simulink model "neural_hopper_wetrace_TD"  (R2018a)
settings: Solver=ode45  StartTime=0.0  StopTime=20  RelTol=1e-4  AbsTol=1e-6  EnableMultiTasking=on
values from neighbouring files (symbols this model uses):
  a = 10    [neural_hopper_wetrace_ISO_params.m]    (also in neural_hopper_wetrace_TD_params.m; neural_hopper_wetrace_params.m)
  b = 10    [neural_hopper_wetrace_ISO_params.m]    (also in neural_hopper_wetrace_TD_params.m; neural_hopper_wetrace_params.m)
  bE = 2.5    [neural_hopper_diff_hebb_params.m]    (also in neural_hopper_params.m = 0.1; neural_hopper_wetrace_ISO_params.m = 0.1; neural_hopper_wetrace_TD_params.m = 0.1; neural_hopper_wetrace_params.m = 0.1)
  c = 0.05    [neural_hopper_diff_hebb_params.m]    (also in neural_hopper_params.m; neural_hopper_wetrace_ISO_params.m; neural_hopper_wetrace_TD_params.m; neural_hopper_wetrace_params.m)
  c_w_F = 0.15    [neural_hopper_wetrace_ISO_params.m]    (also in neural_hopper_wetrace_TD_params.m)
  c_w_l = 0.15    [neural_hopper_wetrace_ISO_params.m]    (also in neural_hopper_wetrace_TD_params.m)
  c_w_v = 0.15    [neural_hopper_wetrace_ISO_params.m]    (also in neural_hopper_wetrace_TD_params.m)
  dy0 = 0    [neural_hopper_diff_hebb_params.m]    (also in neural_hopper_params.m; neural_hopper_wetrace_ISO_params.m; neural_hopper_wetrace_TD_params.m; neural_hopper_wetrace_params.m)
  eref = 0.04    [neural_hopper_diff_hebb_params.m]    (also in neural_hopper_params.m; neural_hopper_wetrace_ISO_params.m; neural_hopper_wetrace_TD_params.m; neural_hopper_wetrace_params.m)
  FmaxVAS = 22000    [neural_hopper_diff_hebb_params.m]    (also in neural_hopper_params.m; neural_hopper_wetrace_ISO_params.m; neural_hopper_wetrace_TD_params.m; neural_hopper_wetrace_params.m)
  g = 9.81    [neural_hopper_diff_hebb_params.m]    (also in neural_hopper_params.m; neural_hopper_wetrace_ISO_params.m; neural_hopper_wetrace_TD_params.m; neural_hopper_wetrace_params.m)
  G_F = 1/(N*FmaxVAS)    (= 3.0303030303e-05)    [neural_hopper_diff_hebb_params.m]    (also in neural_hopper_params.m; neural_hopper_wetrace_ISO_params.m; neural_hopper_wetrace_TD_params.m; neural_hopper_wetrace_params.m)
  G_l = 1/loptVAS    (= 10)    [neural_hopper_diff_hebb_params.m]    (also in neural_hopper_params.m; neural_hopper_wetrace_ISO_params.m = 5; neural_hopper_wetrace_TD_params.m = 5; neural_hopper_wetrace_params.m)
  G_v = -1/(vmaxVAS*loptVAS)    (= -0.833333333333)    [neural_hopper_diff_hebb_params.m]    (also in neural_hopper_params.m; neural_hopper_wetrace_ISO_params.m = -0.416666666667; neural_hopper_wetrace_TD_params.m = -0.416666666667; neural_hopper_wetrace_params.m)
  K = 5    [neural_hopper_diff_hebb_params.m]    (also in neural_hopper_params.m; neural_hopper_wetrace_ISO_params.m; neural_hopper_wetrace_TD_params.m; neural_hopper_wetrace_params.m)
  K_F_et = 200    [neural_hopper_wetrace_ISO_params.m]    (also in neural_hopper_wetrace_TD_params.m; neural_hopper_wetrace_params.m)
  K_l_et = 200    [neural_hopper_wetrace_ISO_params.m]    (also in neural_hopper_wetrace_TD_params.m; neural_hopper_wetrace_params.m)
  K_v_et = 200    [neural_hopper_wetrace_ISO_params.m]    (also in neural_hopper_wetrace_TD_params.m; neural_hopper_wetrace_params.m)
  l0 = 0.99    [neural_hopper_diff_hebb_params.m]    (also in neural_hopper_params.m = 0.9; neural_hopper_wetrace_ISO_params.m; neural_hopper_wetrace_TD_params.m; neural_hopper_wetrace_params.m = 0.9)
  loptVAS = 0.1    [neural_hopper_diff_hebb_params.m]    (also in neural_hopper_params.m; neural_hopper_wetrace_ISO_params.m; neural_hopper_wetrace_TD_params.m; neural_hopper_wetrace_params.m)
  ls = 0.5    [neural_hopper_diff_hebb_params.m]    (also in neural_hopper_params.m; neural_hopper_wetrace_ISO_params.m; neural_hopper_wetrace_TD_params.m; neural_hopper_wetrace_params.m)
  lslackVAS = 0.4    [neural_hopper_diff_hebb_params.m]    (also in neural_hopper_params.m; neural_hopper_wetrace_ISO_params.m; neural_hopper_wetrace_TD_params.m; neural_hopper_wetrace_params.m)
  lVAS0 = loptVAS+lslackVAS    (= 0.5)    [neural_hopper_diff_hebb_params.m]    (also in neural_hopper_params.m; neural_hopper_wetrace_ISO_params.m; neural_hopper_wetrace_TD_params.m; neural_hopper_wetrace_params.m)
  m = 80    [neural_hopper_diff_hebb_params.m]    (also in neural_hopper_params.m; neural_hopper_wetrace_ISO_params.m; neural_hopper_wetrace_TD_params.m; neural_hopper_wetrace_params.m)
  N = 1.5    [neural_hopper_diff_hebb_params.m]    (also in neural_hopper_params.m; neural_hopper_wetrace_ISO_params.m; neural_hopper_wetrace_TD_params.m; neural_hopper_wetrace_params.m)
  r0 = 0.05    [neural_hopper_diff_hebb_params.m]    (also in neural_hopper_params.m; neural_hopper_wetrace_ISO_params.m; neural_hopper_wetrace_TD_params.m; neural_hopper_wetrace_params.m)
  tau = 0.01    [neural_hopper_diff_hebb_params.m]    (also in neural_hopper_params.m; neural_hopper_wetrace_ISO_params.m; neural_hopper_wetrace_TD_params.m; neural_hopper_wetrace_params.m)
  tau_E = 12    [neural_hopper_diff_hebb_params.m]    (also in neural_hopper_params.m; neural_hopper_wetrace_ISO_params.m; neural_hopper_wetrace_TD_params.m; neural_hopper_wetrace_params.m)
  tauE = 0.01    [neural_hopper_diff_hebb_params.m]    (also in neural_hopper_params.m; neural_hopper_wetrace_ISO_params.m; neural_hopper_wetrace_TD_params.m; neural_hopper_wetrace_params.m)
  tauW = 50    [neural_hopper_diff_hebb_params.m]    (also in neural_hopper_params.m = 0.1; neural_hopper_wetrace_ISO_params.m = 0.01; neural_hopper_wetrace_TD_params.m = 0.035; neural_hopper_wetrace_params.m = 0.1)
  theta_u = zeros(3,1)    [neural_hopper_diff_hebb_params.m]    (also in neural_hopper_params.m; neural_hopper_wetrace_ISO_params.m = [0;0;0;0]; neural_hopper_wetrace_TD_params.m = [0;0;0]; neural_hopper_wetrace_params.m)
  thetak0 = 110*pi/180    (= 1.91986217719)    [neural_hopper_diff_hebb_params.m]    (also in neural_hopper_params.m; neural_hopper_wetrace_ISO_params.m; neural_hopper_wetrace_TD_params.m; neural_hopper_wetrace_params.m)
  v_offset = 0    [neural_hopper_wetrace_ISO_params.m]    (also in neural_hopper_wetrace_TD_params.m)
  vmaxVAS = 12    [neural_hopper_diff_hebb_params.m]    (also in neural_hopper_params.m; neural_hopper_wetrace_ISO_params.m; neural_hopper_wetrace_TD_params.m; neural_hopper_wetrace_params.m)
  w = 0.4    [neural_hopper_diff_hebb_params.m]    (also in neural_hopper_params.m; neural_hopper_wetrace_ISO_params.m; neural_hopper_wetrace_TD_params.m; neural_hopper_wetrace_params.m)
  w_F_0 = w_f(3)    [neural_hopper_diff_hebb_params.m]    (also in neural_hopper_params.m = 1; neural_hopper_wetrace_ISO_params.m = 1; neural_hopper_wetrace_TD_params.m = 1; neural_hopper_wetrace_params.m)
  w_F_upper = 4    [neural_hopper_wetrace_ISO_params.m]    (also in neural_hopper_wetrace_TD_params.m)
  w_l_0 = w_f(1)    [neural_hopper_diff_hebb_params.m]    (also in neural_hopper_params.m = 1; neural_hopper_wetrace_ISO_params.m = 1; neural_hopper_wetrace_TD_params.m = 1; neural_hopper_wetrace_params.m)
  w_l_upper = 4    [neural_hopper_wetrace_ISO_params.m]    (also in neural_hopper_wetrace_TD_params.m)
  w_v_0 = w_f(2)    [neural_hopper_diff_hebb_params.m]    (also in neural_hopper_params.m = 1; neural_hopper_wetrace_ISO_params.m = 1; neural_hopper_wetrace_TD_params.m = 1; neural_hopper_wetrace_params.m)
  w_v_upper = 4    [neural_hopper_wetrace_ISO_params.m]    (also in neural_hopper_wetrace_TD_params.m)
  y0 = l0+0.2    (= 1.19)    [neural_hopper_diff_hebb_params.m]    (also in neural_hopper_params.m = 1.1; neural_hopper_wetrace_ISO_params.m; neural_hopper_wetrace_TD_params.m; neural_hopper_wetrace_params.m = 1.1)
libraries: simulink_extras x2, simulink x1
settings Model: Creator=hgeyer  LastModifiedBy=ashwin
settings SolverCC: AutoScaleAbsTol=off
settings DataIOCC: LimitDataPoints=on  SaveFormat=Array  SignalLoggingSaveFormat=ModelDataLogs
settings OptimizationCC: ExpressionDepthLimit=2147483647  LifeSpan=inf
settings DebuggingCC: UnderspecifiedInitializationDetection=Classic  MergeDetectMultiDrivingBlocksExec=none  SolverPrmCheckMsg=warning  FcnCallInpInsideContextMsg=warning  StateNameClashWarn=warning  SFUnexpectedBacktrackingDiag=warning  SFNoUnconditionalDefaultTransitionDiag=warning  SFExecutionAtInitializationDiag=none
settings HardwareCC: ProdBitPerPointer=32  ProdBitPerSizeT=32  ProdBitPerPtrDiffT=32  ProdLargestAtomicFloat=None  ProdIntDivRoundTo=Undefined  ProdEndianess=Unspecified  ProdWordSize=32  ProdHWDeviceType=32-bit Generic
settings ModelReferenceCC: PropagateSignalLabelsOutOfModel=off
settings CodeAppCC: StateflowObjectComments=on
settings GRTTargetCC: TargetLangStandard=C89/C90 (ANSI)  GeneratePreprocessorConditionals=Disable all
settings ConfigComp: CovMetricSettings=dw  CovHtmlReporting=on  CovSaveCumulativeToWorkspaceVar=on  CovSaveSingleToWorkspaceVar=on  CovExternalEMLEnable=off

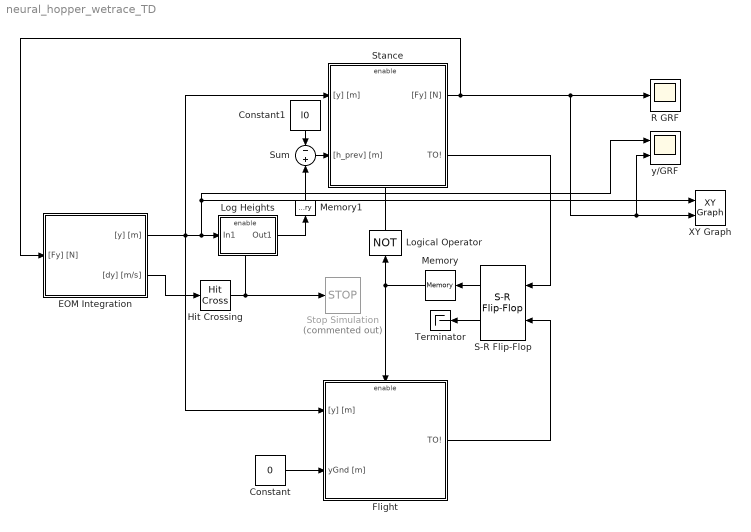
== system neural_hopper_wetrace_TD ==
  Constant : Constant  Value=0
  Constant1 : Constant  Value=l0
  EOM Integration : Subsystem
  Flight : Subsystem
  Hit Crossing : HitCross  HitCrossingDirection=falling
  Log Heights : Subsystem
  Logical Operator : Logic  Operator=NOT  AllPortsSameDT=off  OutDataTypeStr=boolean
  Memory : Memory  InitialCondition=1
  Memory1 : Memory  InitialCondition=y0
  R GRF : Scope
  S-R Flip-Flop : simulink_extras/Flip Flops/S-R Flip-Flop  initial_condition=1
  Stance : Subsystem
  Stop Simulation : Stop  Commented=on
  Sum : Sum  Inputs=-+
  Terminator : Terminator
  XY Graph : simulink/Sinks/XY Graph  xmin=0.6  xmax=1  ymin=0  ymax=5000  st=-1
  "y/GRF " : Scope  NumInputPorts=2
  wires:
  EOM Integration/1("[y] [m]") -> Log Heights/1(In1), "y/GRF "/1, XY Graph/1, Flight/1("[y] [m]"), Stance/1("[y] [m]")
  Stance/2(TO!) -> S-R Flip-Flop/1
  S-R Flip-Flop/1 -> Memory/1
  Logical Operator/1 -> Stance/Enable
  Memory/1 -> Logical Operator/1, Flight/Enable
  Flight/1(TO!) -> S-R Flip-Flop/2
  S-R Flip-Flop/2 -> Terminator/1
  Stance/1("[Fy] [N]") -> "y/GRF "/2, XY Graph/2, R GRF/1, EOM Integration/1("[Fy] [N]")
  Constant/1 -> Flight/2(yGnd [m])
  EOM Integration/2("[dy] [m/s]") -> Hit Crossing/1
  Hit Crossing/1 -> Stop Simulation/1, Log Heights/Enable
  Sum/1 -> Stance/2("[h_prev] [m]")
  Log Heights/1(Out1) -> Memory1/1
  Constant1/1 -> Sum/1
  Memory1/1 -> Sum/2

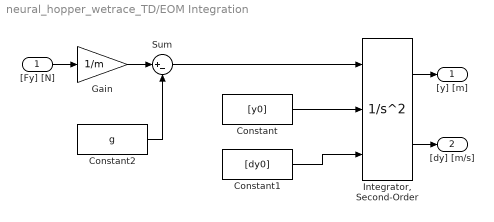
== system neural_hopper_wetrace_TD/EOM Integration ==
  "[Fy] [N]" : Inport
  Constant : Constant  Value=[y0]
  Constant1 : Constant  Value=[dy0]
  Constant2 : Constant  Value=g
  Gain : Gain  Gain=1/m
  "Integrator, Second-Order" : SecondOrderIntegrator  ICSourceX=external  ICSourceDXDT=external
  Sum : Sum  Inputs=|+-
  "[y] [m]" : Outport
  "[dy] [m/s]" : Outport  Port=2
  wires:
  Constant/1 -> "Integrator, Second-Order"/2
  Constant1/1 -> "Integrator, Second-Order"/3
  Gain/1 -> Sum/1
  Sum/1 -> "Integrator, Second-Order"/1
  Constant2/1 -> Sum/2
  "[Fy] [N]"/1 -> Gain/1
  "Integrator, Second-Order"/1 -> "[y] [m]"/1
  "Integrator, Second-Order"/2 -> "[dy] [m/s]"/1

== system neural_hopper_wetrace_TD/Flight ==
  "[y] [m]" : Inport
  yGnd [m] : Inport  Port=2
  Enable : EnablePort  StatesWhenEnabling=reset
  Hit Crossing : HitCross  HitCrossingOffset=l0  HitCrossingDirection=falling
  Sum2 : Sum  Inputs=|+-
  TO! : Outport  OutputWhenDisabled=reset  InitialOutput=0
  wires:
  Hit Crossing/1 -> TO!/1
  "[y] [m]"/1 -> Sum2/1
  yGnd [m]/1 -> Sum2/2
  Sum2/1 -> Hit Crossing/1

== system neural_hopper_wetrace_TD/Log Heights ==
  In1 : Inport
  Enable : EnablePort
  To Workspace : ToWorkspace  VariableName=y_f  SampleTime=-1
  Out1 : Outport
  wires:
  In1/1 -> Out1/1, To Workspace/1

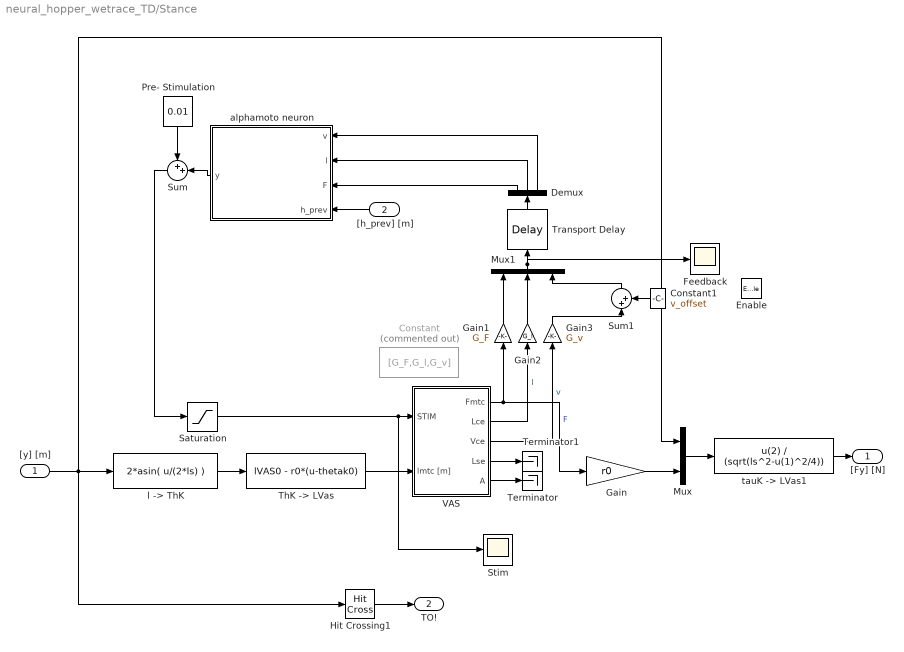
== system neural_hopper_wetrace_TD/Stance ==
  "[y] [m]" : Inport
  "[h_prev] [m]" : Inport  Port=2
  Enable : EnablePort
  Constant : Constant  Commented=on  Value=[G_F,G_l,G_v]  VectorParams1D=off
  Constant1 : Constant  Value=v_offset
  Demux : Demux  Outputs=3
  Feedback : Scope
  Gain : Gain  Gain=r0
  Gain1 : Gain  Gain=G_F
  Gain2 : Gain  Gain=G_l
  Gain3 : Gain  Gain=G_v
  Hit Crossing1 : HitCross  HitCrossingOffset=l0  HitCrossingDirection=rising
  Mux : Mux  Inputs=2
  Mux1 : Mux  Inputs=3
  Pre- Stimulation : Constant  Value=0.01
  Saturation : Saturate  UpperLimit=1  LowerLimit=0.01
  Stim : Scope
  Sum : Sum  Inputs=++|
  Sum1 : Sum  Inputs=|++
  Terminator : Terminator
  Terminator1 : Terminator
  "ThK -> LVas" : Fcn  Expr=lVAS0 - r0*(u-thetak0)
  Transport Delay : TransportDelay  DelayTime=0.01  InitialOutput=[0 0 0]
  VAS : Subsystem
  alphamoto neuron : Subsystem
  "l -> ThK" : Fcn  Expr=2*asin( u/(2*ls) )
  "tauK -> LVas1" : Fcn  Expr=u(2) / (sqrt(ls^2-u(1)^2/4))
  "[Fy] [N]" : Outport  OutputWhenDisabled=reset  InitialOutput=0
  TO! : Outport  Port=2  OutputWhenDisabled=reset  InitialOutput=0
  wires:
  "[y] [m]"/1 -> Mux/1, "l -> ThK"/1, Hit Crossing1/1
  Hit Crossing1/1 -> TO!/1
  "l -> ThK"/1 -> "ThK -> LVas"/1
  "ThK -> LVas"/1 -> VAS/2(lmtc [m])
  Gain/1 -> Mux/2
  Mux/1 -> "tauK -> LVas1"/1
  "tauK -> LVas1"/1 -> "[Fy] [N]"/1
  VAS/1(Fmtc) -> Gain/1, Gain1/1  "F"
  Pre- Stimulation/1 -> Sum/1
  Saturation/1 -> Stim/1, VAS/1(STIM)
  Sum/1 -> Saturation/1
  alphamoto neuron/1(y) -> Sum/2
  VAS/2(Lce) -> Gain2/1  "l"
  Demux/1 -> alphamoto neuron/3(F)
  Demux/2 -> alphamoto neuron/2(l)
  Demux/3 -> alphamoto neuron/1(v)
  Transport Delay/1 -> Demux/1
  VAS/5(A) -> Terminator/1
  VAS/4(Lse) -> Terminator1/1
  Constant1/1 -> Sum1/2
  "[h_prev] [m]"/1 -> alphamoto neuron/4(h_prev)
  VAS/3(Vce) -> Gain3/1  "v"
  Gain3/1 -> Sum1/1
  Gain2/1 -> Mux1/2
  Gain1/1 -> Mux1/1
  Mux1/1 -> Feedback/1, Transport Delay/1
  Sum1/1 -> Mux1/3

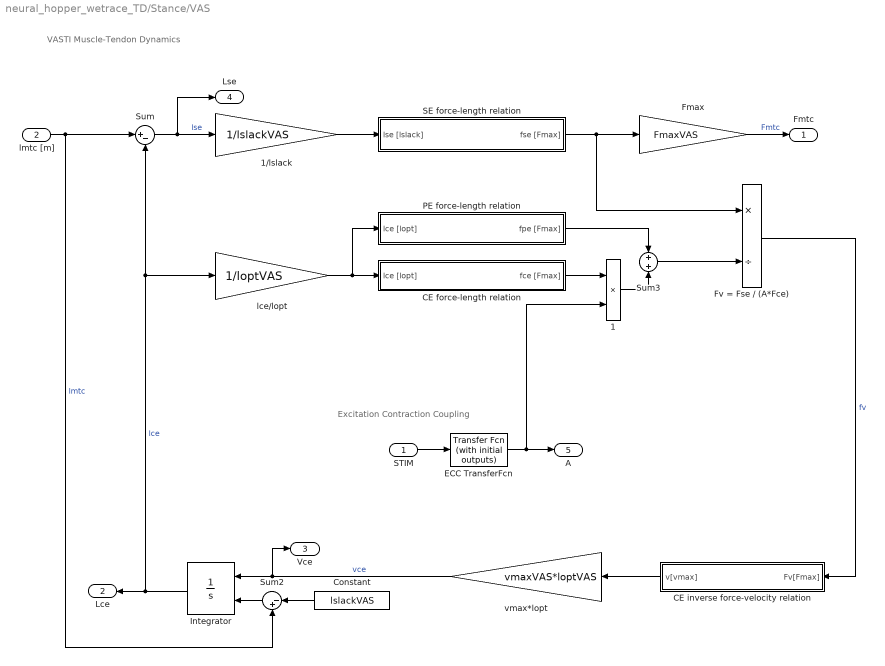
== system neural_hopper_wetrace_TD/Stance/VAS ==
  note: VASTI Muscle-Tendon Dynamics
  note: Excitation Contraction Coupling
  STIM : Inport
  lmtc [m] : Inport  Port=2
  1 : Product  Inputs=**  SaturateOnIntegerOverflow=on  InputSameDT=on  OutDataTypeStr=Inherit: Same as first input
  1/lslack : Gain  Gain=1/lslackVAS  SaturateOnIntegerOverflow=on  OutDataTypeStr=Inherit: Same as input  ParamDataTypeStr=Inherit: Same as input
  CE force-length relation : Subsystem
  CE inverse force-velocity relation : Subsystem
  Constant : Constant  Value=lslackVAS
  ECC TransferFcn : simulink_extras/Additional Linear/Transfer Fcn (with initial outputs)  N=[1]  D="[tau  1]"  Y0=preA  U0=0
      settings: AttributesFormatString=pre-activation: %<Y0>
  Fmax : Gain  Gain=FmaxVAS  SaturateOnIntegerOverflow=on  OutDataTypeStr=Inherit: Same as input  ParamDataTypeStr=Inherit: Same as input
  Fv = Fse / (A*Fce) : Product  Inputs=*/  SaturateOnIntegerOverflow=on  InputSameDT=on  OutDataTypeStr=Inherit: Same as first input
  Integrator : Integrator  InitialConditionSource=external  LowerSaturationLimit=0.05
  PE force-length relation : Subsystem
  SE force-length relation : Subsystem
  Sum : Sum  Inputs=|+-  SaturateOnIntegerOverflow=on  InputSameDT=on  OutDataTypeStr=Inherit: Same as first input
  Sum2 : Sum  Inputs=|-+  SaturateOnIntegerOverflow=on  InputSameDT=on  OutDataTypeStr=Inherit: Same as first input
  Sum3 : Sum  SaturateOnIntegerOverflow=on  InputSameDT=on  OutDataTypeStr=Inherit: Same as first input
  lce/lopt : Gain  Gain=1/loptVAS  SaturateOnIntegerOverflow=on  OutDataTypeStr=Inherit: Same as input  ParamDataTypeStr=Inherit: Same as input
  vmax*lopt : Gain  Gain=vmaxVAS*loptVAS  SaturateOnIntegerOverflow=on  OutDataTypeStr=Inherit: Same as input  ParamDataTypeStr=Inherit: Same as input
  Fmtc : Outport  InitialOutput=0
  Lce : Outport  Port=2  InitialOutput=0
  Vce : Outport  Port=3  InitialOutput=0
  Lse : Outport  Port=4  InitialOutput=0
  A : Outport  Port=5  InitialOutput=0
  wires:
  Integrator/1 -> Sum/2, lce/lopt/1, Lce/1  "lce"
  Sum/1 -> 1/lslack/1, Lse/1  "lse"
  lce/lopt/1 -> CE force-length relation/1(lce [lopt]), PE force-length relation/1(lce [lopt])
  Fv = Fse / (A*Fce)/1 -> CE inverse force-velocity relation/1(Fv[Fmax])  "fv"
  vmax*lopt/1 -> Integrator/1, Vce/1  "vce"
  lmtc [m]/1 -> Sum2/2, Sum/1  "lmtc"
  Fmax/1 -> Fmtc/1  "Fmtc"
  1/lslack/1 -> SE force-length relation/1(lse [lslack])
  Sum2/1 -> Integrator/2
  Constant/1 -> Sum2/1
  CE force-length relation/1(fce [Fmax]) -> 1/1
  SE force-length relation/1(fse [Fmax]) -> Fv = Fse / (A*Fce)/1, Fmax/1
  PE force-length relation/1(fpe [Fmax]) -> Sum3/1
  1/1 -> Sum3/2
  Sum3/1 -> Fv = Fse / (A*Fce)/2
  CE inverse force-velocity relation/1(v[vmax]) -> vmax*lopt/1
  STIM/1 -> ECC TransferFcn/1
  ECC TransferFcn/1 -> 1/2, A/1

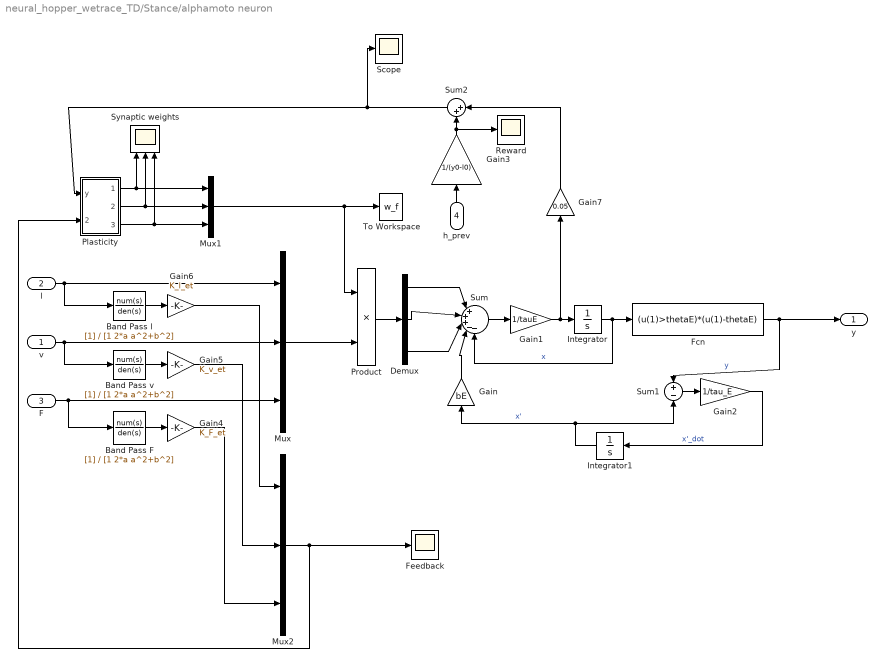
== system neural_hopper_wetrace_TD/Stance/alphamoto neuron ==
  v : Inport
  l : Inport  Port=2
  F : Inport  Port=3
  h_prev : Inport  Port=4
  Band Pass F : TransferFcn  Denominator=[1 2*a a^2+b^2]
  Band Pass l : TransferFcn  Denominator=[1 2*a a^2+b^2]
  Band Pass v : TransferFcn  Denominator=[1 2*a a^2+b^2]
  Demux : Demux  Outputs=3
  Fcn : Fcn  Expr=(u(1)>thetaE)*(u(1)-thetaE)
  Feedback : Scope
  Gain : Gain  Gain=bE
  Gain1 : Gain  Gain=1/tauE
  Gain2 : Gain  Gain=1/tau_E
  Gain3 : Gain  Gain=1/(y0-l0)
  Gain4 : Gain  Gain=K_F_et
  Gain5 : Gain  Gain=K_v_et
  Gain6 : Gain  Gain=K_l_et
  Gain7 : Gain  Gain=0.05
  Integrator : Integrator  InitialCondition=0.01
  Integrator1 : Integrator
  Mux : Mux  Inputs=3
  Mux1 : Mux  Inputs=3
  Mux2 : Mux  Inputs=3
  Plasticity : Subsystem
  Product : Product
  Reward : Scope
  Scope : Scope
  Sum : Sum  Inputs=|+++--
  Sum1 : Sum  Inputs=+-
  Sum2 : Sum  Inputs=|++
  Synaptic weights : Scope  NumInputPorts=3
  To Workspace : ToWorkspace  VariableName=w_f  SampleTime=-1
  y : Outport
  wires:
  Integrator1/1 -> Gain/1, Sum1/2  "x'"
  Gain/1 -> Sum/4
  Sum1/1 -> Gain2/1
  Gain2/1 -> Integrator1/1  "x'_dot"
  Gain1/1 -> Gain7/1, Integrator/1
  Sum/1 -> Gain1/1
  Fcn/1 -> y/1, Sum1/1  "y"
  Integrator/1 -> Sum/5, Fcn/1  "x"
  Demux/1 -> Sum/1
  Demux/3 -> Sum/3
  Demux/2 -> Sum/2
  v/1 -> Mux/2, Band Pass v/1
  l/1 -> Mux/1, Band Pass l/1
  F/1 -> Band Pass F/1, Mux/3
  Mux1/1 -> Product/1, To Workspace/1
  Product/1 -> Demux/1
  Plasticity/3(w_F) -> Mux1/3, Synaptic weights/3
  Plasticity/2(w_l) -> Mux1/2, Synaptic weights/2
  Plasticity/1(w_v) -> Synaptic weights/1, Mux1/1
  Band Pass F/1 -> Gain4/1
  Band Pass v/1 -> Gain5/1
  Band Pass l/1 -> Gain6/1
  Gain6/1 -> Mux2/1
  Gain5/1 -> Mux2/2
  Gain4/1 -> Mux2/3
  Mux2/1 -> Plasticity/2(In2), Feedback/1
  Mux/1 -> Product/2
  h_prev/1 -> Gain3/1
  Sum2/1 -> Scope/1, Plasticity/1(y)
  Gain3/1 -> Reward/1, Sum2/2
  Gain7/1 -> Sum2/1

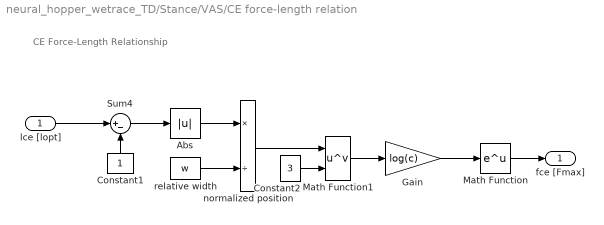
== system neural_hopper_wetrace_TD/Stance/VAS/CE force-length relation ==
  note: CE Force-Length Relationship
  lce [lopt] : Inport
  Abs : Abs
  Constant1 : Constant
  Constant2 : Constant  Value=3
  Gain : Gain  Gain=log(c)
  Math Function : Math  SaturateOnIntegerOverflow=on
  Math Function1 : Math  Operator=pow  SaturateOnIntegerOverflow=on
  Sum4 : Sum  Inputs=|+-  SaturateOnIntegerOverflow=on  InputSameDT=on  OutDataTypeStr=Inherit: Same as first input
  normalized position : Product  Inputs=*/
  relative width : Constant  Value=w
  fce [Fmax] : Outport
  wires:
  lce [lopt]/1 -> Sum4/1
  relative width/1 -> normalized position/2
  Constant1/1 -> Sum4/2
  Sum4/1 -> Abs/1
  Abs/1 -> normalized position/1
  normalized position/1 -> Math Function1/1
  Constant2/1 -> Math Function1/2
  Math Function1/1 -> Gain/1
  Gain/1 -> Math Function/1
  Math Function/1 -> fce [Fmax]/1

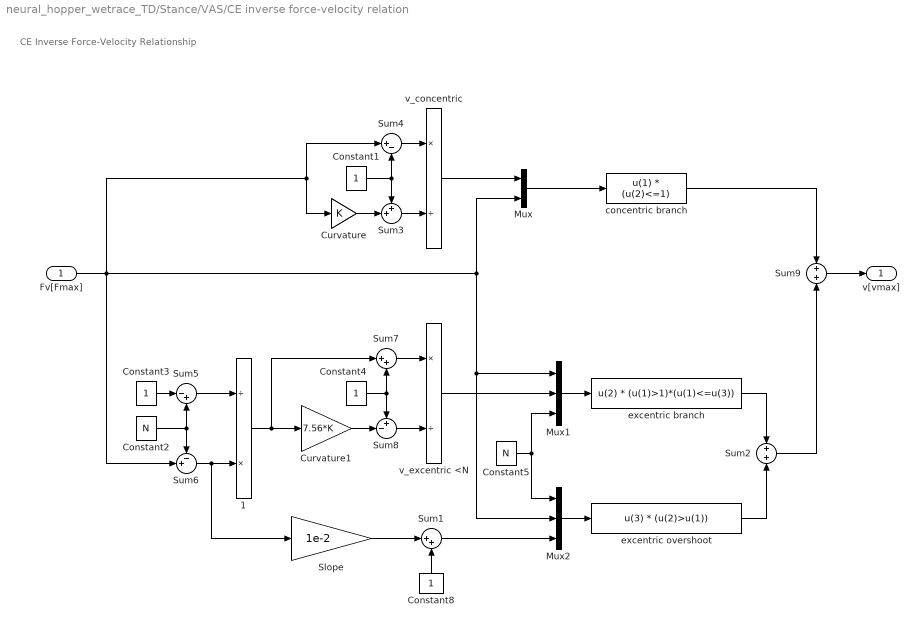
== system neural_hopper_wetrace_TD/Stance/VAS/CE inverse force-velocity relation ==
  note: CE Inverse Force-Velocity Relationship
  Fv[Fmax] : Inport
  1 : Product  Inputs=/*
  Constant{1,3..4,8} (4 alike) : Constant
  Constant2 : Constant  Value=N
  Constant5 : Constant  Value=N
  Curvature : Gain  Gain=K  SaturateOnIntegerOverflow=on  OutDataTypeStr=Inherit: Same as input  ParamDataTypeStr=Inherit: Same as input
  Curvature1 : Gain  Gain=7.56*K  SaturateOnIntegerOverflow=on  OutDataTypeStr=Inherit: Same as input  ParamDataTypeStr=Inherit: Same as input
  Mux : Mux  Inputs=2
  Mux1 : Mux  Inputs=3
  Mux2 : Mux  Inputs=3
  Slope : Gain  Gain=1e-2  SaturateOnIntegerOverflow=on  OutDataTypeStr=Inherit: Same as input  ParamDataTypeStr=Inherit: Same as input
  Sum1 : Sum  Inputs=|++  SaturateOnIntegerOverflow=on  InputSameDT=on  OutDataTypeStr=Inherit: Same as first input
  Sum2 : Sum  SaturateOnIntegerOverflow=on  InputSameDT=on  OutDataTypeStr=Inherit: Same as first input
  Sum3 : Sum  Inputs=++|  SaturateOnIntegerOverflow=on  InputSameDT=on  OutDataTypeStr=Inherit: Same as first input
  Sum4 : Sum  Inputs=|+-  SaturateOnIntegerOverflow=on  InputSameDT=on  OutDataTypeStr=Inherit: Same as first input
  Sum5 : Sum  Inputs=|-+  SaturateOnIntegerOverflow=on  InputSameDT=on  OutDataTypeStr=Inherit: Same as first input
  Sum6 : Sum  Inputs=-+|  SaturateOnIntegerOverflow=on  InputSameDT=on  OutDataTypeStr=Inherit: Same as first input
  Sum7 : Sum  Inputs=|++  SaturateOnIntegerOverflow=on  InputSameDT=on  OutDataTypeStr=Inherit: Same as first input
  Sum8 : Sum  Inputs=+-|  SaturateOnIntegerOverflow=on  InputSameDT=on  OutDataTypeStr=Inherit: Same as first input
  Sum9 : Sum  SaturateOnIntegerOverflow=on  InputSameDT=on  OutDataTypeStr=Inherit: Same as first input
  concentric branch : Fcn  Expr=u(1) * (u(2)<=1)
  excentric branch : Fcn  Expr=u(2) * (u(1)>1)*(u(1)<=u(3))
  excentric overshoot : Fcn  Expr=u(3) * (u(2)>u(1))
  v_concentric : Product  Inputs=*/
  v_excentric <N : Product  Inputs=*/
  v[vmax] : Outport
  wires:
  Curvature/1 -> Sum3/2
  Constant1/1 -> Sum4/2, Sum3/1
  Sum4/1 -> v_concentric/1
  Sum3/1 -> v_concentric/2
  1/1 -> Sum7/1, Curvature1/1
  Constant4/1 -> Sum7/2, Sum8/1
  Curvature1/1 -> Sum8/2
  Sum8/1 -> v_excentric <N/2
  Sum7/1 -> v_excentric <N/1
  v_concentric/1 -> Mux/1
  Fv[Fmax]/1 -> Sum4/1, Curvature/1, Sum6/2, Mux/2, Mux1/1, Mux2/2
  Sum9/1 -> v[vmax]/1
  Sum2/1 -> Sum9/2
  excentric overshoot/1 -> Sum2/2
  Slope/1 -> Sum1/1
  Constant8/1 -> Sum1/2
  Sum6/1 -> 1/2, Slope/1
  Constant2/1 -> Sum6/1, Sum5/2
  Sum5/1 -> 1/1
  Constant3/1 -> Sum5/1
  Mux/1 -> concentric branch/1
  Mux1/1 -> excentric branch/1
  v_excentric <N/1 -> Mux1/2
  Mux2/1 -> excentric overshoot/1
  concentric branch/1 -> Sum9/1
  excentric branch/1 -> Sum2/1
  Constant5/1 -> Mux1/3, Mux2/1
  Sum1/1 -> Mux2/3

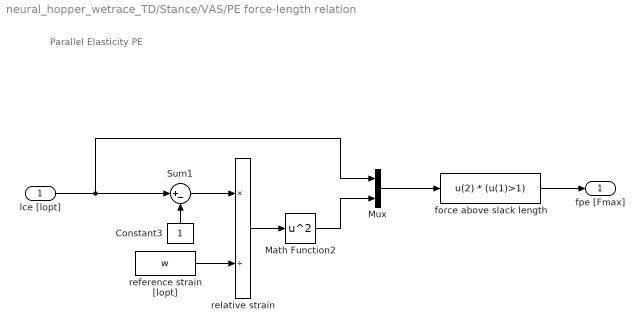
== system neural_hopper_wetrace_TD/Stance/VAS/PE force-length relation ==
  note: Parallel Elasticity PE
  lce [lopt] : Inport
  Constant3 : Constant
  Math Function2 : Math  Operator=square  SaturateOnIntegerOverflow=on
  Mux : Mux  Inputs=2
  Sum1 : Sum  Inputs=|+-  SaturateOnIntegerOverflow=on  InputSameDT=on  OutDataTypeStr=Inherit: Same as first input
  force above slack length : Fcn  Expr=u(2) * (u(1)>1)
  reference strain [lopt] : Constant  Value=w
  relative strain : Product  Inputs=*/
  fpe [Fmax] : Outport
  wires:
  Mux/1 -> force above slack length/1
  lce [lopt]/1 -> Mux/1, Sum1/1
  Constant3/1 -> Sum1/2
  Sum1/1 -> relative strain/1
  reference strain [lopt]/1 -> relative strain/2
  relative strain/1 -> Math Function2/1
  Math Function2/1 -> Mux/2
  force above slack length/1 -> fpe [Fmax]/1

== system neural_hopper_wetrace_TD/Stance/VAS/SE force-length relation ==
  note: SE Force-Length Relationship
  lse [lslack] : Inport
  Constant1 : Constant
  Math Function : Math  Operator=square  SaturateOnIntegerOverflow=on
  Mux : Mux  Inputs=2
  Sum4 : Sum  Inputs=|+-  SaturateOnIntegerOverflow=on  InputSameDT=on  OutDataTypeStr=Inherit: Same as first input
  force above slack length : Fcn  Expr=u(2)*(u(1)>1)
  reference strain [lslack] : Constant  Value=eref
  relative strain : Product  Inputs=*/
  fse [Fmax] : Outport
  wires:
  Mux/1 -> force above slack length/1
  force above slack length/1 -> fse [Fmax]/1
  Math Function/1 -> Mux/2
  lse [lslack]/1 -> Mux/1, Sum4/1
  relative strain/1 -> Math Function/1
  reference strain [lslack]/1 -> relative strain/2
  Sum4/1 -> relative strain/1
  Constant1/1 -> Sum4/2

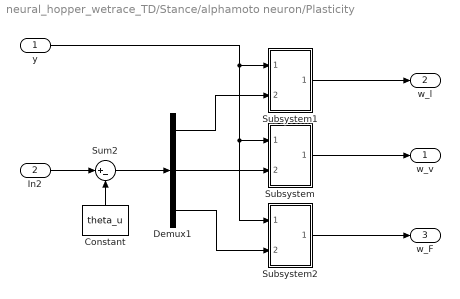
== system neural_hopper_wetrace_TD/Stance/alphamoto neuron/Plasticity ==
  y : Inport
  In2 : Inport  Port=2
  Constant : Constant  Value=theta_u
  Demux1 : Demux  Outputs=3
  Subsystem : Subsystem
  Subsystem1 : Subsystem
  Subsystem2 : Subsystem
  Sum2 : Sum  Inputs=|+-
  w_v : Outport
  w_l : Outport  Port=2
  w_F : Outport  Port=3
  wires:
  In2/1 -> Sum2/1
  Constant/1 -> Sum2/2
  Sum2/1 -> Demux1/1
  Subsystem/1(w_v) -> w_v/1
  Demux1/2 -> Subsystem/2(In2)
  Demux1/1 -> Subsystem1/2(In2)
  Subsystem1/1(w_l) -> w_l/1
  y/1 -> Subsystem1/1(In1), Subsystem/1(In1), Subsystem2/1(In1)
  Demux1/3 -> Subsystem2/2(In2)
  Subsystem2/1(w_F) -> w_F/1

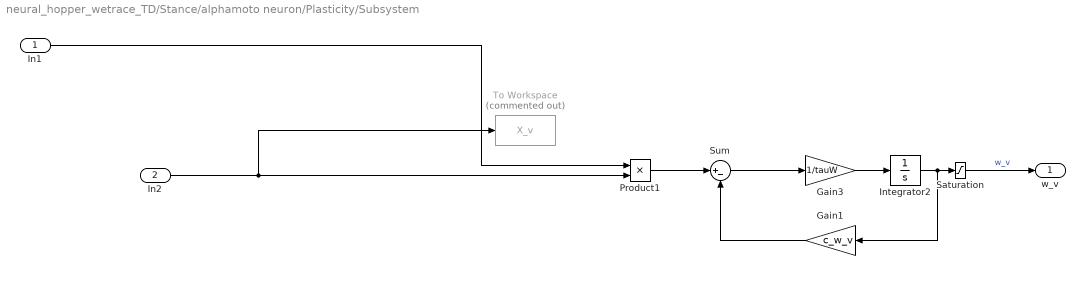
== system neural_hopper_wetrace_TD/Stance/alphamoto neuron/Plasticity/Subsystem ==
  In1 : Inport
  In2 : Inport  Port=2
  Gain1 : Gain  Gain=c_w_v
  Gain3 : Gain  Gain=1/tauW
  Integrator2 : Integrator  InitialCondition=w_v_0
  Product1 : Product
  Saturation : Saturate  UpperLimit=w_v_upper  LowerLimit=0.01
  Sum : Sum  Inputs=|+-
  To Workspace : ToWorkspace  Commented=on  VariableName=X_v  SampleTime=-1
      settings: MaxDataPoints=window_  Save2DSignal=2-D array (concatenate along first dimension)
  w_v : Outport
  wires:
  Saturation/1 -> w_v/1  "w_v"
  In2/1 -> Product1/2, To Workspace/1
  Integrator2/1 -> Gain1/1, Saturation/1
  In1/1 -> Product1/1
  Product1/1 -> Sum/1
  Sum/1 -> Gain3/1
  Gain1/1 -> Sum/2
  Gain3/1 -> Integrator2/1

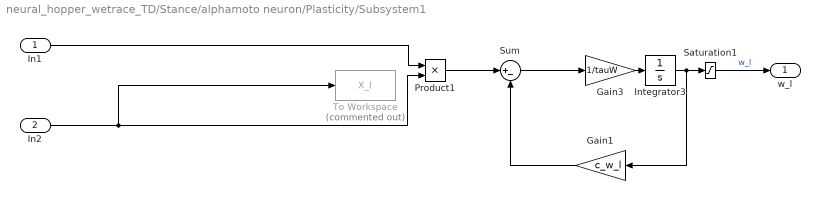
== system neural_hopper_wetrace_TD/Stance/alphamoto neuron/Plasticity/Subsystem1 ==
  In1 : Inport
  In2 : Inport  Port=2
  Gain1 : Gain  Gain=c_w_l
  Gain3 : Gain  Gain=1/tauW
  Integrator3 : Integrator  InitialCondition=w_l_0
  Product1 : Product
  Saturation1 : Saturate  UpperLimit=w_l_upper  LowerLimit=0.01
  Sum : Sum  Inputs=|+-
  To Workspace : ToWorkspace  Commented=on  VariableName=X_l  SampleTime=-1
      settings: MaxDataPoints=window_  Save2DSignal=2-D array (concatenate along first dimension)
  w_l : Outport
  wires:
  In2/1 -> Product1/2, To Workspace/1
  In1/1 -> Product1/1
  Saturation1/1 -> w_l/1  "w_l"
  Integrator3/1 -> Gain1/1, Saturation1/1
  Gain3/1 -> Integrator3/1
  Sum/1 -> Gain3/1
  Product1/1 -> Sum/1
  Gain1/1 -> Sum/2

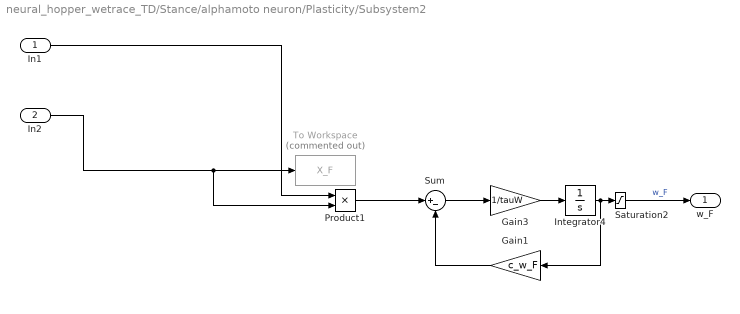
== system neural_hopper_wetrace_TD/Stance/alphamoto neuron/Plasticity/Subsystem2 ==
  In1 : Inport
  In2 : Inport  Port=2
  Gain1 : Gain  Gain=c_w_F
  Gain3 : Gain  Gain=1/tauW
  Integrator4 : Integrator  InitialCondition=w_F_0
  Product1 : Product
  Saturation2 : Saturate  UpperLimit=w_F_upper  LowerLimit=0.01
  Sum : Sum  Inputs=|+-
  To Workspace : ToWorkspace  Commented=on  VariableName=X_F  SampleTime=-1
      settings: MaxDataPoints=window_  Save2DSignal=2-D array (concatenate along first dimension)
  w_F : Outport
  wires:
  In1/1 -> Product1/1
  In2/1 -> Product1/2, To Workspace/1
  Saturation2/1 -> w_F/1  "w_F"
  Product1/1 -> Sum/1
  Sum/1 -> Gain3/1
  Gain1/1 -> Sum/2
  Gain3/1 -> Integrator4/1
  Integrator4/1 -> Gain1/1, Saturation2/1
